simulink model "ThreePhase_3Level_Converter_Hysteresis_Control"  (R2022a)
settings: Solver=VariableStepAuto  StartTime=0.0  StopTime=0.2  MaxStep=1e-5  RelTol=1e-3
libraries: spsMosfetLib x12, spsCurrentMeasurementLib x8, spsDiodeLib x6, spsSeriesRLCBranchLib x5, spsGroundLib x4, spsPLL3phLib x2, eePowerMeasurement x2, spsThreePhaseProgrammableVoltageSourceLib x2, spsThreePhaseVIMeasurementLib x2, spsDCVoltageSourceLib x2, spsVoltageMeasurementLib x2, spsThreePhaseSeriesRLCLoadLib x1
settings Model: Creator=Vigneshwaran R  LastModifiedBy=hp

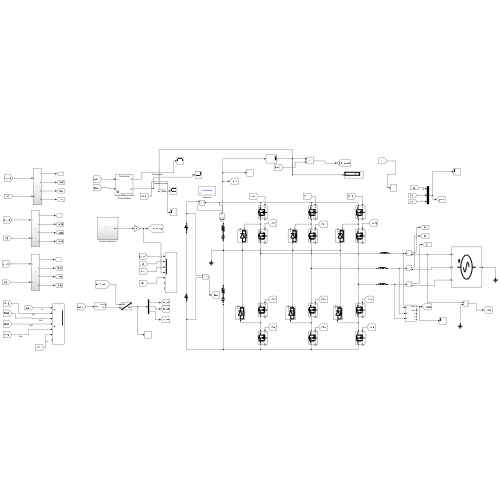
[thumbnail: Simulink's stored preview of the top-level diagram]
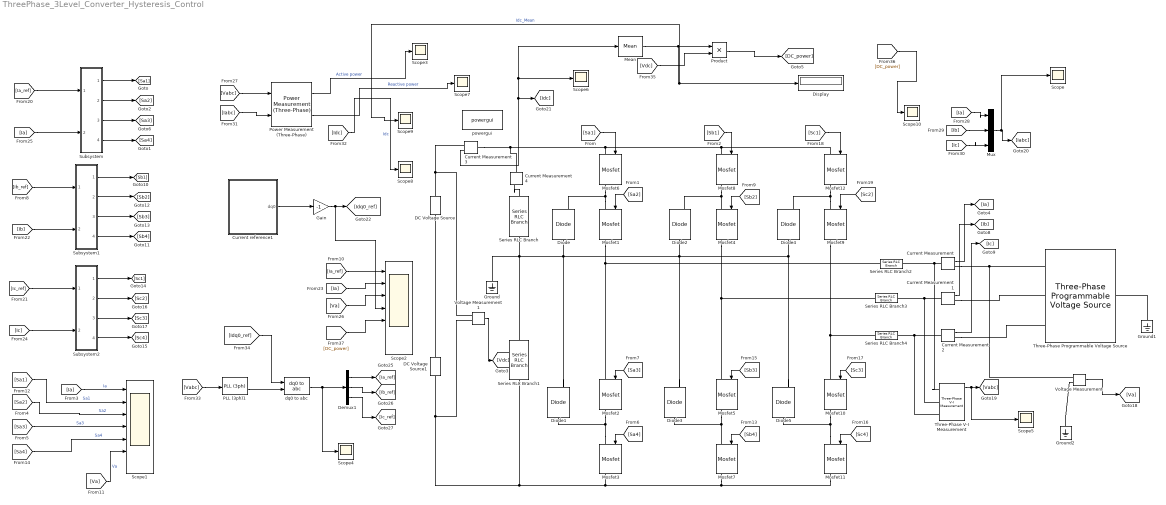
== system ThreePhase_3Level_Converter_Hysteresis_Control ==
  Current Measurement{,1..4} (5 alike) : spsCurrentMeasurementLib/Current Measurement  PhasorSimulation=off  OutputType=Complex  PSBequivalent=0
  Current reference1 : Subsystem
  DC Voltage Source : spsDCVoltageSourceLib/DC Voltage Source  Amplitude=300  Measurements=None
  DC Voltage Source1 : spsDCVoltageSourceLib/DC Voltage Source  Amplitude=300  Measurements=None
  Demux1 : Demux  Outputs=3
  Diode{,1..5} (6 alike) : spsDiodeLib/Diode  Ron=0.001  Lon=0  Vf=0.8  IC=0  UseSnubber=0  Rs=500  Cs=250e-9  Measurements=on
  Display : Display
  Gain : Gain  Gain=-1
  Ground : spsGroundLib/Ground  LConnTagsString=a
  Ground1 : spsGroundLib/Ground  LConnTagsString=a
  Ground2 : spsGroundLib/Ground  LConnTagsString=a
  Mean : spsMeanLib/Mean  Freq=50  Vinit=0  Ts=0
  Mosfet{1..12} (12 alike) : spsMosfetLib/Mosfet  Ron=0.1  Lon=0  Rd=0.01  Vfd=0  IC=0  Rs=1e5  Cs=inf  Measurements=on
  Mux : Mux  Inputs=3
  PLL (3ph)1 : spsPLL3phLib/PLL (3ph)  Fmin=45  Par_Init=[-90, 50]  ParK=[180, 3200, 1]  TcD=1e-4  MaxRateChangeFreq=12  FilterCutOffFreq=25  Ts=0  AGC=on
  Power Measurement (Three-Phase) : eePowerMeasurement/Power Measurement (Three-Phase)  LabelModeActiveChoice=Continuous  F=50  K=[1]  Seq=Positive  Ts=0
      settings: SourceProductBaseCode=PS
  Product : Product
  Scope{,3..10} (9 alike) : Scope
  Scope1 : Scope  NumInputPorts=7
  Scope2 : Scope  NumInputPorts=7
  Series RLC Branch : spsSeriesRLCBranchLib/Series RLC Branch  LConnTagsString=__new0  RConnTagsString=__new0  BranchType=RC  Resistance=0.1  Inductance=1e-3  SetiL0=off  InitialCurrent=0  Capacitance=6e-6  Setx0=off  InitialVoltage=0  Measurements=None
  Series RLC Branch1 : spsSeriesRLCBranchLib/Series RLC Branch  LConnTagsString=__new0  RConnTagsString=__new0  BranchType=RC  Resistance=0.1  Inductance=1e-3  SetiL0=off  InitialCurrent=0  Capacitance=6e-6  Setx0=off  InitialVoltage=0  Measurements=None
  Series RLC Branch2 : spsSeriesRLCBranchLib/Series RLC Branch  LConnTagsString=__new0  RConnTagsString=__new0  BranchType=L  Resistance=5  Inductance=8.06e-3  SetiL0=off  InitialCurrent=0  Capacitance=1e-6  Setx0=off  InitialVoltage=0  Measurements=None
  Series RLC Branch3 : spsSeriesRLCBranchLib/Series RLC Branch  LConnTagsString=__new0  RConnTagsString=__new0  BranchType=L  Resistance=5  Inductance=8.06e-3  SetiL0=off  InitialCurrent=0  Capacitance=1e-6  Setx0=off  InitialVoltage=0  Measurements=None
  Series RLC Branch4 : spsSeriesRLCBranchLib/Series RLC Branch  LConnTagsString=__new0  RConnTagsString=__new0  BranchType=L  Resistance=5  Inductance=8.06e-3  SetiL0=off  InitialCurrent=0  Capacitance=1e-6  Setx0=off  InitialVoltage=0  Measurements=None
  Subsystem : Subsystem
  Subsystem1 : Subsystem
  Subsystem2 : Subsystem
  Three-Phase Programmable Voltage Source : spsThreePhaseProgrammableVoltageSourceLib/Three-Phase Programmable Voltage Source  PositiveSequence="[415  0 50]"  VariationEntity=None  VariationType=Table of time-amplitude pairs  VariationTypeAlt=Step  VariationStep=0.5  VariationRate=10  VariationMagnitude=0.3  VariationFrequency=2  VariationTiming=[1 2]  VariationPhaseA=off  Amplitudes=[1 0.8 1.2 1.0]  TimeValues=[0 0.1 0.15 0.2]  HarmonicGeneration=off  HarmonicA=[3 0.2 -25 0]  HarmonicB=[2 0.15 35 2]  Timing="[0.05  3]"  BusType=swing  Pref=0  Qref=0  Qmin=-inf  Qmax=inf
  Three-Phase V-I Measurement : spsThreePhaseVIMeasurementLib/Three-Phase V-I Measurement  VoltageMeasurement=phase-to-ground  SetLabelV=off  LabelV=Vabc  Vpu=off  VpuLL=off  CurrentMeasurement=yes  SetLabelI=off  LabelI=Iabc  Ipu=off  Pbase=100e6  Vbase=500e3  OutputType=Complex  PhasorSimulation=off  PSBequivalent=0
  Voltage Measurement : spsVoltageMeasurementLib/Voltage Measurement  PhasorSimulation=off  OutputType=Complex  PSBequivalent=0
  Voltage Measurement1 : spsVoltageMeasurementLib/Voltage Measurement  PhasorSimulation=off  OutputType=Complex  PSBequivalent=0
  dq0 to abc : spsdq0toabcLib/dq0 to abc  Alignment=90 degrees behind phase A axis
  powergui : spspowerguiLib/powergui  Priority=1  SimulationMode=Continuous  SampleTime=50e-6  frequency=60  Iterations=50  frequencyindice=50  Pbase=100e6  ErrMax=1e-4  UnitsV=kV  UnitsW=MW  buscounter=0  FunctionMessages=off  echomessages=off  EnableUseOfTLC=off  CurrentSourceSwitches=off  DisableSnubberDevices=off  DisableRonSwitches=off  DisableVfSwitches=off  DisplayEquations=off  AutomaticDiscreteSolvers=off  SolverType=Tustin/Backward Euler (TBE)  Interpol=off  ExternalGateDelay=off  methode=off  Ts=100  x0status=blocks  SPID=on  SwTol=0  HookPort=off  NonlinearTolerance=1e-4  nMaxIteration=100  ContinueOnMaxIteration=off  RestoreLinks=warning  ResistiveCurrentMeasurement=off  Frange=[0:2:500]  Ylog=off  Xlog=on  ShowGrid=off  save=off  variable=ZData  structure=0  ZoomFFT=off  StartTime=0.0  cycles=1  DisplayStyle=1  fundamental=60  FreqAxis=off  MaxFrequency=1000  frequencyindicesteady=1  RmsSteady=1  display=off
  wires:
  [Sa2] -> Mosfet1/1
  [Sa4] -> Mosfet3/1
  [Sa2] -> Scope1/3  "Sa2"
  [Sa3] -> Scope1/4  "Sa3"
  [Sa3] -> Mosfet2/1
  [Ia] -> Scope1/1  "Ia"
  [Sa1] -> Mosfet6/1
  [Ia_ref] -> Scope2/1
  [Sa4] -> Scope1/5  "Sa4"
  [Sa1] -> Scope1/2  "Sa1"
  Subsystem/1(Out1) -> [Sa1]
  Subsystem/2(Out2) -> [Sa2]
  Subsystem/3(Out3) -> [Sa3]
  Subsystem/4(Out4) -> [Sa4]
  [Sb1] -> Mosfet8/1
  [Sb3] -> Mosfet5/1
  [Sb4] -> Mosfet7/1
  [Sb2] -> Mosfet4/1
  [Sc2] -> Mosfet9/1
  [Sc4] -> Mosfet11/1
  [Sc3] -> Mosfet10/1
  [Sc1] -> Mosfet12/1
  Current reference1/1(dq0) -> Gain/1
  Gain/1 -> Scope2/4, [Idq0_ref]
  [Ia_ref] -> Subsystem/1(In1)
  Current Measurement/1 -> [Ia]
  Current Measurement1/1 -> [Ib]
  Current Measurement2/1 -> [Ic]
  Subsystem1/4(Out4) -> [Sb4]
  Subsystem1/3(Out3) -> [Sb3]
  Subsystem1/2(Out2) -> [Sb2]
  Subsystem1/1(Out1) -> [Sb1]
  [Ic] -> Subsystem2/2(In2)
  Subsystem2/1(Out1) -> [Sc1]
  Subsystem2/2(Out2) -> [Sc2]
  Subsystem2/3(Out3) -> [Sc3]
  Subsystem2/4(Out4) -> [Sc4]
  [Ic_ref] -> Subsystem2/1(In1)
  [Ia] -> Subsystem/2(In2)
  [Ib_ref] -> Subsystem1/1(In1)
  [Ib] -> Subsystem1/2(In2)
  Voltage Measurement/1 -> [Va]
  [Va] -> Scope1/6  "Va"
  [Ia] -> Scope2/2
  [Va] -> Scope2/3
  Power Measurement (Three-Phase)/1 -> Scope3/1  "Active power"
  Power Measurement (Three-Phase)/2 -> Scope7/1  "Reactive power"
  Three-Phase V-I Measurement/1 -> Scope5/1, [Vabc]
  [Vabc] -> Power Measurement (Three-Phase)/1
  [Ia] -> Mux/1
  [Ib] -> Mux/2
  [Ic] -> Mux/3
  Mux/1 -> Scope/1, [Iabc]
  [Iabc] -> Power Measurement (Three-Phase)/2
  Current Measurement3/1 -> Mean/1, Scope6/1, [Idc]
  [Idc] -> Scope8/1  "Idc"
  [Vabc] -> PLL (3ph)1/1
  [Idq0_ref] -> dq0 to abc/1
  PLL (3ph)1/2 -> dq0 to abc/2
  dq0 to abc/1 -> Scope4/1, Demux1/1
  Demux1/1 -> [Ia_ref]
  Demux1/2 -> [Ib_ref]
  Demux1/3 -> [Ic_ref]
  Voltage Measurement1/1 -> [Vdc]
  Mean/1 -> Scope9/1, Display/1, Product/1  "Idc_Mean"
  [Vdc] -> Product/2
  Product/1 -> [DC_power]
  [DC_power] -> Scope10/1
  [DC_power] -> Scope2/5
  connections:
  Current Measurement3/LConn1 -- Mosfet8/LConn1 -- Mosfet12/LConn1 -- Mosfet6/LConn1 -- Current Measurement4/LConn1
  Mosfet3/LConn1 -- Mosfet2/RConn1 -- Diode1/LConn1
  Mosfet1/RConn1 -- Series RLC Branch2/LConn1 -- Mosfet2/LConn1
  Mosfet1/LConn1 -- Mosfet6/RConn1 -- Diode/RConn1
  DC Voltage Source1/LConn1 -- Voltage Measurement1/LConn2 -- Series RLC Branch1/RConn1 -- Mosfet7/RConn1 -- Mosfet11/RConn1 -- Mosfet3/RConn1
  Mosfet5/RConn1 -- Mosfet7/LConn1 -- Diode3/LConn1
  Mosfet8/RConn1 -- Mosfet4/LConn1 -- Diode2/RConn1
  Mosfet4/RConn1 -- Series RLC Branch3/LConn1 -- Mosfet5/LConn1
  Mosfet11/LConn1 -- Mosfet10/RConn1 -- Diode5/LConn1
  Mosfet9/LConn1 -- Mosfet12/RConn1 -- Diode4/RConn1
  Mosfet9/RConn1 -- Series RLC Branch4/LConn1 -- Mosfet10/LConn1
  Current Measurement/LConn1 -- Three-Phase V-I Measurement/LConn1 -- Series RLC Branch2/RConn1
  Current Measurement1/LConn1 -- Three-Phase V-I Measurement/LConn2 -- Series RLC Branch3/RConn1
  Current Measurement2/LConn1 -- Three-Phase V-I Measurement/LConn3 -- Series RLC Branch4/RConn1
  Current Measurement/RConn1 -- Voltage Measurement/LConn1 -- Three-Phase Programmable Voltage Source/RConn1
  Current Measurement1/RConn1 -- Three-Phase Programmable Voltage Source/RConn2
  Current Measurement2/RConn1 -- Three-Phase Programmable Voltage Source/RConn3
  Ground1/LConn1 -- Three-Phase Programmable Voltage Source/LConn1
  Ground2/LConn1 -- Voltage Measurement/LConn2
  Voltage Measurement1/LConn1 -- DC Voltage Source/RConn1 -- Current Measurement3/RConn1
  Diode4/LConn1 -- Ground/LConn1 -- Series RLC Branch1/LConn1 -- Series RLC Branch/RConn1 -- Diode1/RConn1 -- Diode/LConn1 -- Diode2/LConn1 -- Diode3/RConn1 -- Diode5/RConn1
  Current Measurement4/RConn1 -- Series RLC Branch/LConn1
  DC Voltage Source1/RConn1 -- DC Voltage Source/LConn1

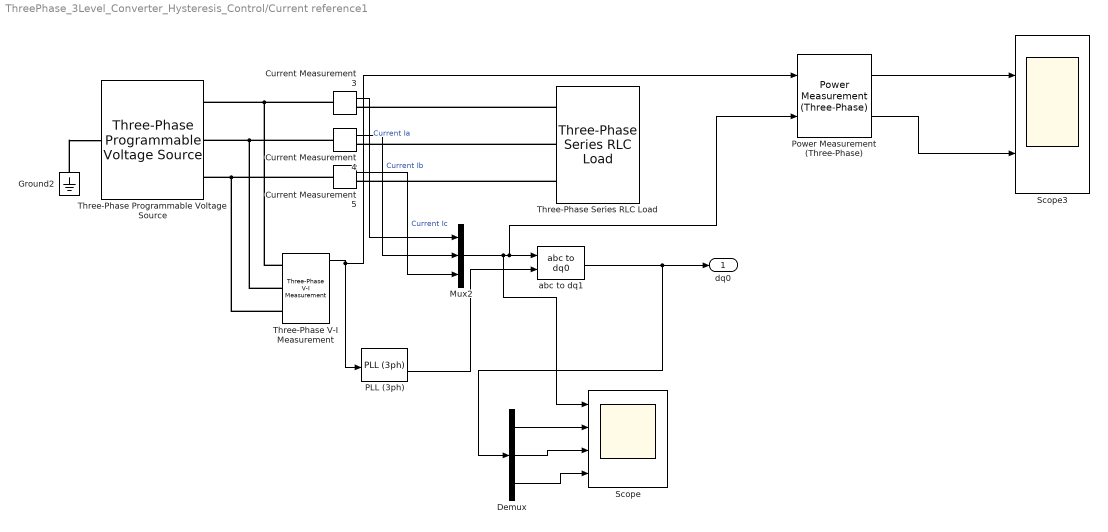
== system ThreePhase_3Level_Converter_Hysteresis_Control/Current reference1 ==
  Current Measurement3 : spsCurrentMeasurementLib/Current Measurement  PhasorSimulation=off  OutputType=Complex  PSBequivalent=0
  Current Measurement4 : spsCurrentMeasurementLib/Current Measurement  PhasorSimulation=off  OutputType=Complex  PSBequivalent=0
  Current Measurement5 : spsCurrentMeasurementLib/Current Measurement  PhasorSimulation=off  OutputType=Complex  PSBequivalent=0
  Demux : Demux  Outputs=3
  Ground2 : spsGroundLib/Ground  LConnTagsString=a
  Mux2 : Mux  Inputs=3
  PLL (3ph) : spsPLL3phLib/PLL (3ph)  Fmin=45  Par_Init=[0, 60]  ParK=[180, 3200, 1]  TcD=1e-4  MaxRateChangeFreq=12  FilterCutOffFreq=25  Ts=0  AGC=on
  Power Measurement (Three-Phase) : eePowerMeasurement/Power Measurement (Three-Phase)  LabelModeActiveChoice=Continuous  F=50  K=[1]  Seq=Positive  Ts=0
      settings: SourceProductBaseCode=PS
  Scope : Scope  NumInputPorts=4
  Scope3 : Scope  NumInputPorts=2
  Three-Phase Programmable Voltage Source : spsThreePhaseProgrammableVoltageSourceLib/Three-Phase Programmable Voltage Source  PositiveSequence=[415 0 50]  VariationEntity=None  VariationType=Table of time-amplitude pairs  VariationTypeAlt=Step  VariationStep=0.5  VariationRate=10  VariationMagnitude=0.3  VariationFrequency=2  VariationTiming=[1 2]  VariationPhaseA=off  Amplitudes=[1 0.8 1.2 1.0]  TimeValues=[0 0.1 0.15 0.2]  HarmonicGeneration=off  HarmonicA=[3 0.2 -25 0]  HarmonicB=[2 0.15 35 2]  Timing="[0.05  3]"  BusType=swing  Pref=0  Qref=0  Qmin=-inf  Qmax=inf
  Three-Phase Series RLC Load : spsThreePhaseSeriesRLCLoadLib/Three-Phase Series RLC Load  LConnTagsString=A|B|C  Configuration=Y (grounded)  NominalVoltage=415  Vabc=[1e3 1e3 1e3]  Vabcp=[1e3 1e3 1e3]  NominalFrequency=50  UnbalancedPower=off  ActivePower=10e3  InductivePower=0  CapacitivePower=0  Pabc=[10e3 9e3 11e3]  QLabc=[100 90 110]  QCabc=[100 90 110]  Pabcp=[10e3 9e3 11e3]  QLabcp=[100 90 110]  QCabcp=[100 90 110]  Measurements=None  LoadType=constant Z
  Three-Phase V-I Measurement : spsThreePhaseVIMeasurementLib/Three-Phase V-I Measurement  VoltageMeasurement=phase-to-ground  SetLabelV=off  LabelV=Vabc  Vpu=off  VpuLL=off  CurrentMeasurement=yes  SetLabelI=off  LabelI=Iabc  Ipu=off  Pbase=100e6  Vbase=500e3  OutputType=Complex  PhasorSimulation=off  PSBequivalent=0
  abc to dq1 : spsabctodq0Lib/abc to dq0  Alignment=90 degrees behind phase A axis
  dq0 : Outport
  wires:
  Current Measurement5/1 -> Mux2/3  "Current Ic"
  Current Measurement4/1 -> Mux2/2  "Current Ib"
  Mux2/1 -> Scope/1, Power Measurement (Three-Phase)/2, abc to dq1/1
  Current Measurement3/1 -> Mux2/1  "Current Ia"
  PLL (3ph)/2 -> abc to dq1/2
  abc to dq1/1 -> Demux/1, dq0/1
  Demux/1 -> Scope/2
  Demux/2 -> Scope/3
  Demux/3 -> Scope/4
  Three-Phase V-I Measurement/1 -> Power Measurement (Three-Phase)/1, PLL (3ph)/1
  Power Measurement (Three-Phase)/1 -> Scope3/1
  Power Measurement (Three-Phase)/2 -> Scope3/2
  connections:
  Three-Phase Series RLC Load/LConn3 -- Current Measurement5/RConn1
  Current Measurement3/LConn1 -- Three-Phase V-I Measurement/LConn1 -- Three-Phase Programmable Voltage Source/RConn1
  Ground2/LConn1 -- Three-Phase Programmable Voltage Source/LConn1
  Three-Phase Series RLC Load/LConn1 -- Current Measurement3/RConn1
  Current Measurement4/LConn1 -- Three-Phase V-I Measurement/LConn2 -- Three-Phase Programmable Voltage Source/RConn2
  Current Measurement5/LConn1 -- Three-Phase V-I Measurement/LConn3 -- Three-Phase Programmable Voltage Source/RConn3
  Three-Phase Series RLC Load/LConn2 -- Current Measurement4/RConn1

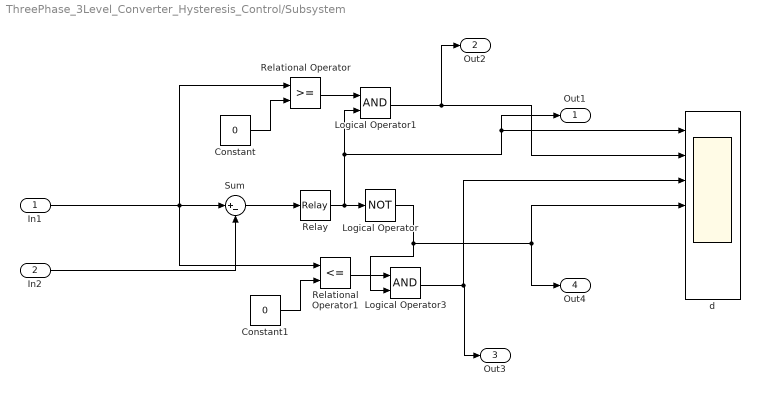
== system ThreePhase_3Level_Converter_Hysteresis_Control/Subsystem ==
  In1 : Inport
  In2 : Inport  Port=2
  Constant : Constant  Value=0
  Constant1 : Constant  Value=0
  Logical Operator : Logic  Operator=NOT  AllPortsSameDT=off  OutDataTypeStr=boolean
  Logical Operator1 : Logic  AllPortsSameDT=off  OutDataTypeStr=boolean
  Logical Operator3 : Logic  AllPortsSameDT=off  OutDataTypeStr=boolean
  Relational Operator : RelationalOperator  OutDataTypeStr=boolean  RndMeth=Simplest  InputSameDT=off
  Relational Operator1 : RelationalOperator  Operator=<=  OutDataTypeStr=boolean  RndMeth=Simplest  InputSameDT=off
  Relay : Relay  OnSwitchValue=1  OffSwitchValue=-1
  Sum : Sum  Inputs=|+-
  d : Scope  NumInputPorts=7
  Out1 : Outport
  Out2 : Outport  Port=2
  Out3 : Outport  Port=3
  Out4 : Outport  Port=4
  wires:
  Relay/1 -> d/1, Out1/1, Logical Operator1/2, Logical Operator/1
  Constant1/1 -> Relational Operator1/2
  Constant/1 -> Relational Operator/2
  Sum/1 -> Relay/1
  Relational Operator/1 -> Logical Operator1/1
  Logical Operator/1 -> Out4/1, d/4, Logical Operator3/2
  Relational Operator1/1 -> Logical Operator3/1
  In1/1 -> Relational Operator1/1, Relational Operator/1, Sum/1
  Logical Operator1/1 -> d/2, Out2/1
  In2/1 -> Sum/2
  Logical Operator3/1 -> d/3, Out3/1

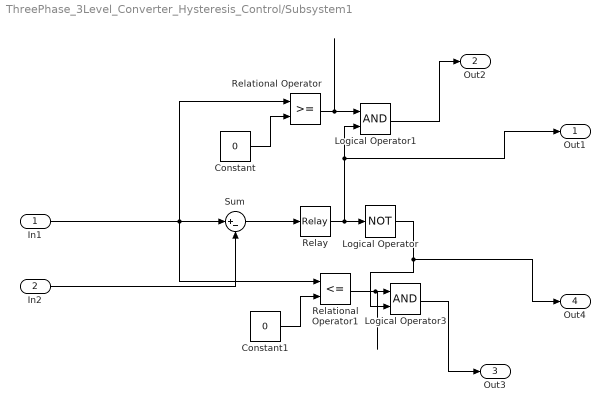
== system ThreePhase_3Level_Converter_Hysteresis_Control/Subsystem1 ==
  In1 : Inport
  In2 : Inport  Port=2
  Constant : Constant  Value=0
  Constant1 : Constant  Value=0
  Logical Operator : Logic  Operator=NOT  AllPortsSameDT=off  OutDataTypeStr=boolean
  Logical Operator1 : Logic  AllPortsSameDT=off  OutDataTypeStr=boolean
  Logical Operator3 : Logic  AllPortsSameDT=off  OutDataTypeStr=boolean
  Relational Operator : RelationalOperator  OutDataTypeStr=boolean  RndMeth=Simplest  InputSameDT=off
  Relational Operator1 : RelationalOperator  Operator=<=  OutDataTypeStr=boolean  RndMeth=Simplest  InputSameDT=off
  Relay : Relay  OnSwitchValue=1  OffSwitchValue=-1
  Sum : Sum  Inputs=|+-
  Out1 : Outport
  Out2 : Outport  Port=2
  Out3 : Outport  Port=3
  Out4 : Outport  Port=4
  wires:
  Logical Operator3/1 -> Out3/1
  In2/1 -> Sum/2
  Logical Operator1/1 -> Out2/1
  In1/1 -> Sum/1, Relational Operator/1, Relational Operator1/1
  Relational Operator1/1 -> Logical Operator3/1
  Logical Operator/1 -> Out4/1, Logical Operator3/2
  Relational Operator/1 -> Logical Operator1/1
  Sum/1 -> Relay/1
  Constant/1 -> Relational Operator/2
  Constant1/1 -> Relational Operator1/2
  Relay/1 -> Logical Operator/1, Out1/1, Logical Operator1/2

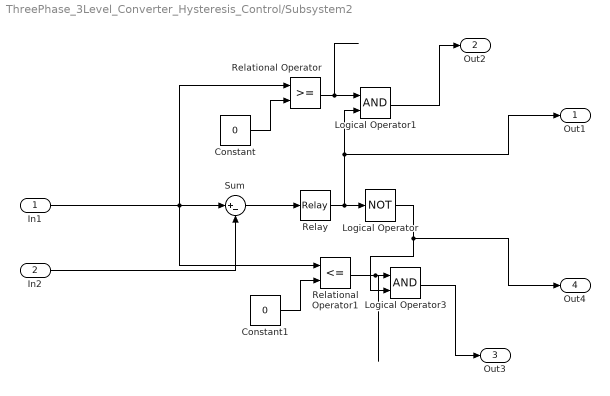
== system ThreePhase_3Level_Converter_Hysteresis_Control/Subsystem2 ==
  In1 : Inport
  In2 : Inport  Port=2
  Constant : Constant  Value=0
  Constant1 : Constant  Value=0
  Logical Operator : Logic  Operator=NOT  AllPortsSameDT=off  OutDataTypeStr=boolean
  Logical Operator1 : Logic  AllPortsSameDT=off  OutDataTypeStr=boolean
  Logical Operator3 : Logic  AllPortsSameDT=off  OutDataTypeStr=boolean
  Relational Operator : RelationalOperator  OutDataTypeStr=boolean  RndMeth=Simplest  InputSameDT=off
  Relational Operator1 : RelationalOperator  Operator=<=  OutDataTypeStr=boolean  RndMeth=Simplest  InputSameDT=off
  Relay : Relay  OnSwitchValue=1  OffSwitchValue=-1
  Sum : Sum  Inputs=|+-
  Out1 : Outport
  Out2 : Outport  Port=2
  Out3 : Outport  Port=3
  Out4 : Outport  Port=4
  wires:
  Logical Operator3/1 -> Out3/1
  In2/1 -> Sum/2
  Logical Operator1/1 -> Out2/1
  In1/1 -> Sum/1, Relational Operator/1, Relational Operator1/1
  Relational Operator1/1 -> Logical Operator3/1
  Relational Operator/1 -> Logical Operator1/1
  Sum/1 -> Relay/1
  Constant/1 -> Relational Operator/2
  Constant1/1 -> Relational Operator1/2
  Relay/1 -> Logical Operator/1, Out1/1, Logical Operator1/2
  Logical Operator/1 -> Out4/1, Logical Operator3/2
